simulink model "motor"  (R2022b)
settings: Solver=ode45  StartTime=0.0  StopTime=18  MaxStep=0.0001  RelTol=1e-3
values from neighbouring files (symbols this model uses):
  input = 3    [ex1.m]
undefined symbols (not defined in the file or in its folder): degs2rpm, diff, National_Instruments, PCIe, pid, rpm2rads, sens, stair, step, triang
libraries: sldrtlib x3, simulink x2
settings Model: Creator=loren  LastModifiedBy=loren
settings DataIOCC: ReturnWorkspaceOutputs=off
settings ModelReferenceCC: EnableRefExpFcnMdlSchedulingChecks=on

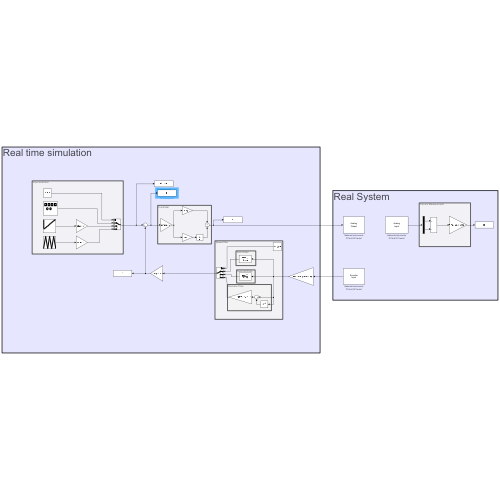
[thumbnail: Simulink's stored preview of the top-level diagram]
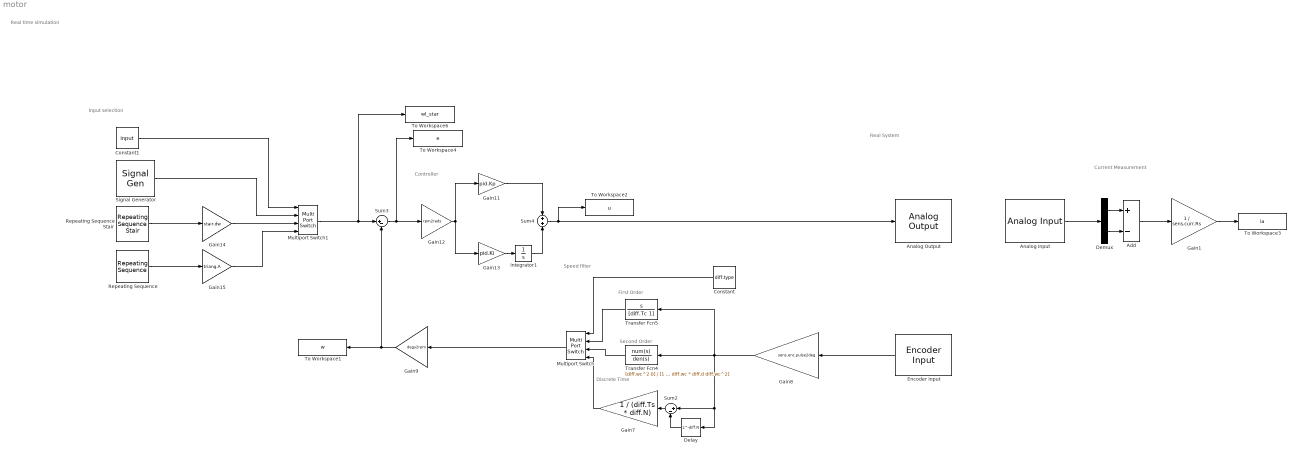
== system motor ==
  note: Current Measurement
  note: Real System
  note: Real time simulation
  note: Input selection
  note: Controller
  note: Speed filter
  note: Discrete Time
  note: Second Order
  note: First Order
  Add : Sum  Inputs=+-
  Analog Input : sldrtlib/Analog Input  SampleTime=-1  MaxMissedTicks=10  ShowMissedTicks=off  YieldWhenWaiting=off  DrvName=National_Instruments/PCIe-6321  DrvAddress=4294967295  DrvOptions=[0 0 0 2 0 0 0]  Channels=[1 2]  RangeMode=1  VoltRange=1  DataType=1
      settings: AttributesFormatString=National Instruments\nPCIe-6321 [auto]
  Analog Output : sldrtlib/Analog Output  SampleTime=-1  MaxMissedTicks=10  ShowMissedTicks=off  YieldWhenWaiting=off  DrvName=National_Instruments/PCIe-6321  DrvAddress=4294967295  DrvOptions=[0 0 0 2 0 0 0]  Channels=1  RangeMode=1  VoltRange=1  InitialValue=0  FinalValue=0
      settings: AttributesFormatString=National Instruments\nPCIe-6321 [auto]
  Constant : Constant  Value=diff.type
  Constant1 : Constant  Value=input
  Delay : Delay  DelayLength=diff.N
  Demux : Demux  Outputs=2
  Encoder Input : sldrtlib/Encoder Input  SampleTime=-1  MaxMissedTicks=10  ShowMissedTicks=off  YieldWhenWaiting=off  DrvName=National_Instruments/PCIe-6321  DrvAddress=4294967295  DrvOptions=[0 0 0 2 0 0 0]  Channels=1  QuadMode=3  IndexPulse=1  InputFilter=Inf  DataType=1
      settings: AttributesFormatString=National Instruments\nPCIe-6321 [auto]
  Gain1 : Gain  Gain=1 / sens.curr.Rs
  Gain11 : Gain  Gain=pid.Kp
  Gain12 : Gain  Gain=rpm2rads
  Gain13 : Gain  Gain=pid.Ki
  Gain14 : Gain  Gain=stair.dw
  Gain15 : Gain  Gain=triang.A
  Gain7 : Gain  Gain=1 / (diff.Ts * diff.N)
  Gain8 : Gain  Gain=sens.enc.pulse2deg
  Gain9 : Gain  Gain=degs2rpm
  Integrator1 : Integrator
  Multiport Switch : MultiPortSwitch  SaturateOnIntegerOverflow=off  InputSameDT=off
  Multiport Switch1 : MultiPortSwitch  SaturateOnIntegerOverflow=off  InputSameDT=off
  Repeating Sequence : simulink/Sources/Repeating Sequence  rep_seq_t=triang.times  rep_seq_y=triang.values
  Repeating Sequence Stair : simulink/Sources/Repeating Sequence Stair  OutValues=stair.k'  tsamp=stair.dt  OutMin=[]  OutMax=[]  OutDataTypeStr=double  OutputDataTypeScalingMode=double  OutDataType=fixdt(0,8)  ConRadixGroup=Best Precision: Vector-wise  OutScaling=2^-12
  Signal Generator : SignalGenerator  WaveForm=square  Amplitude=step.A  Frequency=1 / step.T
  Sum2 : Sum  Inputs=|+-
  Sum3 : Sum  Inputs=|+-
  Sum4 : Sum  Inputs=+|+
  To Workspace1 : ToWorkspace  VariableName=w  SaveFormat=Timeseries  SampleTime=-1
  To Workspace2 : ToWorkspace  VariableName=u  SaveFormat=Timeseries  SampleTime=-1
  To Workspace3 : ToWorkspace  VariableName=ia  SaveFormat=Timeseries  SampleTime=-1
  To Workspace4 : ToWorkspace  VariableName=e  SaveFormat=Timeseries  SampleTime=-1
  To Workspace6 : ToWorkspace  VariableName=wl_star  SaveFormat=Timeseries  SampleTime=-1
  Transfer Fcn4 : TransferFcn  Numerator=[diff.wc^2 0]  Denominator=[1 2 * diff.wc * diff.d diff.wc^2]
  Transfer Fcn5 : TransferFcn  Numerator=[1 0]  Denominator=[diff.Tc 1]
  wires:
  Gain8/1 -> Transfer Fcn5/1, Transfer Fcn4/1, Delay/1, Sum2/1
  Delay/1 -> Sum2/2
  Sum2/1 -> Gain7/1
  Multiport Switch/1 -> Gain9/1
  Transfer Fcn5/1 -> Multiport Switch/2
  Transfer Fcn4/1 -> Multiport Switch/3
  Constant/1 -> Multiport Switch/1
  Gain9/1 -> To Workspace1/1, Sum3/2
  Sum3/1 -> Gain12/1, To Workspace4/1
  Gain12/1 -> Gain11/1, Gain13/1
  Sum4/1 -> Analog Output/1, To Workspace2/1
  Gain11/1 -> Sum4/1
  Gain13/1 -> Integrator1/1
  Integrator1/1 -> Sum4/2
  Gain7/1 -> Multiport Switch/4
  Repeating Sequence Stair/1 -> Gain14/1
  Gain14/1 -> Multiport Switch1/3
  Signal Generator/1 -> Multiport Switch1/2
  Constant1/1 -> Multiport Switch1/1
  Repeating Sequence/1 -> Gain15/1
  Gain15/1 -> Multiport Switch1/4
  Multiport Switch1/1 -> To Workspace6/1, Sum3/1
  Encoder Input/1 -> Gain8/1
  Analog Input/1 -> Demux/1
  Demux/1 -> Add/1
  Demux/2 -> Add/2
  Add/1 -> Gain1/1
  Gain1/1 -> To Workspace3/1
